simulink model "P4semmod_simulink"  (R2025b)
settings: Solver=VariableStepAuto  StartTime=0.0  StopTime=10.0  RelTol=1e-3
settings Model: Creator=raul  LastModifiedBy=raul

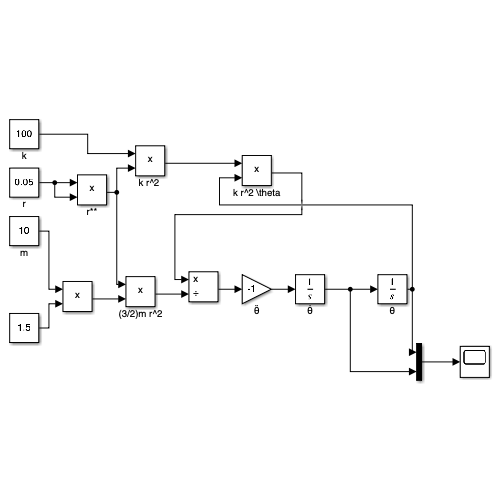
[thumbnail: Simulink's stored preview of the top-level diagram]
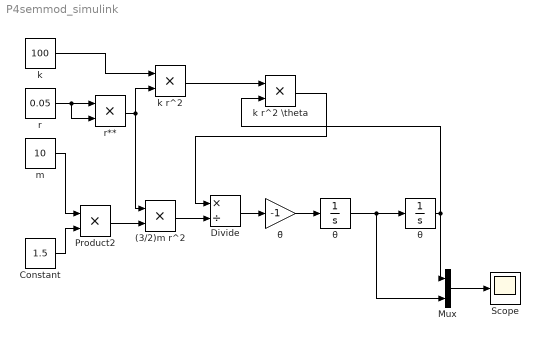
== system P4semmod_simulink ==
  (3/2)m r^2 : Product
  Constant : Constant  Value=1.5
  Divide : Product  Inputs=*/
  Mux : Mux  Inputs=2
  Product2 : Product
  Scope : Scope
      settings: ActiveDisplayYMinimum=-2.4995493874118879  ActiveDisplayYMaximum=2.4999499319346543
  k : Constant  Value=100
  "k r^2 " : Product
  k r^2 \theta : Product
  m : Constant  Value=10
  r : Constant  Value=0.05
  r** : Product
  θ : Integrator
  θ̇ : Integrator  InitialCondition=2
  θ̈ : Gain  Gain=-1
  wires:
  r/1 -> r**/2, r**/1
  r**/1 -> (3/2)m r^2/1, "k r^2 "/2
  k/1 -> "k r^2 "/1
  "k r^2 "/1 -> k r^2 \theta/1
  θ/1 -> Mux/1, k r^2 \theta/2
  m/1 -> Product2/1
  Constant/1 -> Product2/2
  Product2/1 -> (3/2)m r^2/2
  (3/2)m r^2/1 -> Divide/2
  k r^2 \theta/1 -> Divide/1
  Divide/1 -> θ̈/1
  θ̈/1 -> θ̇/1
  θ̇/1 -> Mux/2, θ/1
  Mux/1 -> Scope/1
